simulink model "model2"  (R2022b)
settings: Solver=ode4  StartTime=0.0  StopTime=2  FixedStep=1e-5  RelTol=1e-3
InitFcn:
  | model_
values from neighbouring files (symbols this model uses):
  f = 50    [model_.m]
  J = 0.4    [model_.m]
  pp = 2    [model_.m]
undefined symbols (not defined in the file or in its folder): L1, L1sigma, L2, L2sigma, Lm, R1, R2, sigma
settings Model: Creator=petrzakopal  LastModifiedBy=petrzakopal

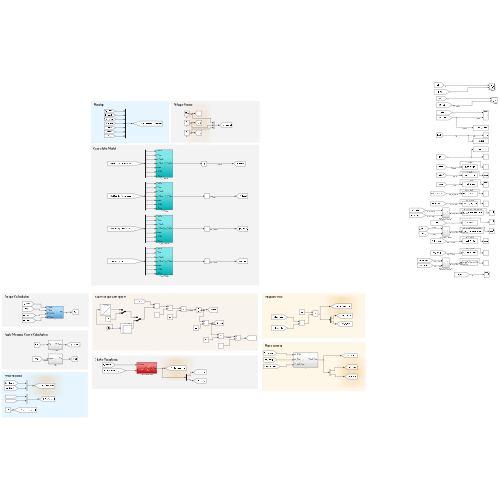
[thumbnail: Simulink's stored preview of the top-level diagram]
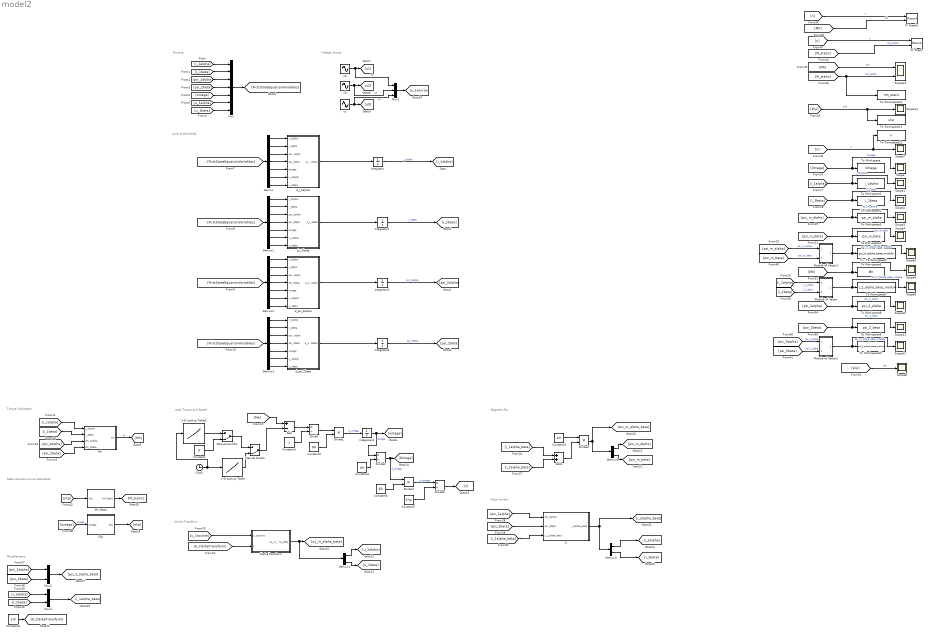
== system model2 ==
  note: Magnetic flux
  note: Rotor current
  note: Load Torque and Speed
  note: Clarke Transform
  note: Static Moment Curve Calculation
  note: Torque Calculation
  note: Core of the Model
  note: Miscellaneous
  note: Routing
  note: Voltage Source
  1-D Lookup Table : Lookup_n-D  NumberOfTableDimensions=1  BreakpointsForDimension1=[0;1.00001;1.001;10]  Table=[0;0;25;25]  InternalRulePriority=Speed  RndMeth=Simplest
  1-D Lookup Table2 : Lookup_n-D  NumberOfTableDimensions=1  BreakpointsForDimension1=[1;2;10]  Table=[0;0;78.48]  InternalRulePriority=Speed  RndMeth=Simplest
  Add : Sum  Inputs=+-
  Add1 : Sum
  ClarkeTransform : Subsystem
  Clock : Clock
  Constant : Constant  Value=0
  Constant1 : Constant  Value=J
  Constant2 : Constant  Value=pp
  Constant3 : Constant  Value=2/3
  Constant4 : Constant  Value=pp
  Constant5 : Constant  Value=Lm
  Constant6 : Constant  Value=60
  Constant7 : Constant  Value=2*pi
  Demux{,1..3} (4 alike) : Demux  Outputs=7
  Demux4 : Demux  Outputs=2
  Demux5 : Demux  Outputs=2
  Demux6 : Demux  Outputs=2
  Divide : Product  Inputs=*/
  Divide1 : Product  Inputs=**
  Divide2 : Product  Inputs=*/
  Divide3 : Product  Inputs=**
  Divide4 : Product  Inputs=**
  Divide5 : Product  Inputs=*/
  Integrator{,1..4} (5 alike) : Integrator
  Manual Switch : ManualSwitch  CurrentSetting=0
  Manual Switch1 : ManualSwitch  CurrentSetting=0
  Mh : Subsystem
  Mh Static : Subsystem
  Module of Vector : Subsystem
  Module of Vector1 : Subsystem
  Module of Vector2 : Subsystem
  Mux : Mux  Inputs=7
  Mux1 : Mux  Inputs=3
  Mux2 : Mux  Inputs=2
  Mux4 : Mux  Inputs=2
  Scope{,1..12,14} (14 alike) : Scope
  Scope13 : Scope  NumInputPorts=2
  Slip : Subsystem
  To Workspace : ToWorkspace  VariableName=Omega  SaveFormat=Timeseries  SampleTime=-1
  To Workspace1 : ToWorkspace  VariableName=i_1alpha  SaveFormat=Timeseries  SampleTime=-1
  To Workspace10 : ToWorkspace  VariableName=psi_2_alpha_beta_module  SaveFormat=Timeseries  SampleTime=-1
  To Workspace11 : ToWorkspace  VariableName=slip  SaveFormat=Timeseries  SampleTime=-1
  To Workspace12 : ToWorkspace  VariableName=mh_static  SaveFormat=Timeseries  SampleTime=-1
  To Workspace13 : ToWorkspace  VariableName=n  SaveFormat=Timeseries  SampleTime=-1
  To Workspace2 : ToWorkspace  VariableName=i_1beta  SaveFormat=Timeseries  SampleTime=-1
  To Workspace3 : ToWorkspace  VariableName=psi_m_alpha  SaveFormat=Timeseries  SampleTime=-1
  To Workspace4 : ToWorkspace  VariableName=psi_m_beta  SaveFormat=Timeseries  SampleTime=-1
  To Workspace5 : ToWorkspace  VariableName=psi_m_alpha_beta_module  SaveFormat=Timeseries  SampleTime=-1
  To Workspace6 : ToWorkspace  VariableName=Mh  SaveFormat=Timeseries  SampleTime=-1
  To Workspace7 : ToWorkspace  VariableName=i_1_alpha_beta_module  SaveFormat=Timeseries  SampleTime=-1
  To Workspace8 : ToWorkspace  VariableName=psi_2_alpha  SaveFormat=Timeseries  SampleTime=-1
  To Workspace9 : ToWorkspace  VariableName=psi_2_beta  SaveFormat=Timeseries  SampleTime=-1
  XY Graph : Record  FileSettingsInternal="{\"entries\":[{\"content\":{\"excelSettings\":{\"content\":{},\"type\":\"Streamout.ExcelSettings\"}},\"type\":\"Streamout.FileSettingStorage\",\"uuid\":\"842da89f-1fef-4ffd-8a1c-7bfb6317d6bb\"}],\"packageUris\":[\"http://schema.mathworks.com/mf0/streamout_blocks/R2020a\"],\"version\":\"1.0\"}"  Layout=[1 1]  SignalsInternal="{\"entries\":[{\"content\":{\"signals\":[{\"content\":{\"blockPath\":[\"model/XY Graph\"],\"channel\":[],\"dimensions\":[1],\"domain\":\"model/XY Graph\",\"lineColor\":\"#a2142f\",\"plots\":[1],\"port\":1,\"sid\":[],\"signalID\":16,\"signalName\":\"n\"},\"type\":\"RecordBlkView.Signal\",\"uuid\":\"3fa61c07-4d6e-48c9-97ec-bc673b73ea1e\"},{\"content\":{\"blockPath\":[\"model/XY Graph\"],\"channel\":[],\"dimensions\":[1],\"domain\":\"model/XY Graph\",\"lineColor\":\"#139fff\",\"plots\":[1],\"port\":2,\"sid\":[],\"signalID\":19,\"signalName\":\"Mh_static\"},\"type\":\"RecordBlkView.Signal\",\"uuid\":\"76ceb205-9b97-4673-bf6a-aa09134c6add\"}]},\"type\":\"RecordBlkView.InputSignals\",\"uuid\":\"48bfde53-39e3-4f40-beb6-cae9881eed94\"}],\"packageUris\":[\"http://schema.mathworks.com/mf0/streamout_blocks/R2020a\"],\"version\":\"1.0\"}"  VisualizationBindings="{\"xyplotplugin\":{\"info\":[{\"series\":[{\"bindingParametersList\":[{\"parameter\":\"X-Axis\",\"signalID\":16,\"signalName\":\"n\"},{\"parameter\":\"Y-Axis\",\"signalID\":19,\"signalName\":\"Mh_static\"}],\"seriesID\":25766}],\"subplotID\":1}]}}"  CompatibilityTag=XY
  XY Graph1 : Record  FileSettingsInternal="{\"entries\":[{\"content\":{\"excelSettings\":{\"content\":{},\"type\":\"Streamout.ExcelSettings\"}},\"type\":\"Streamout.FileSettingStorage\",\"uuid\":\"3db78ad4-fa90-443a-83a0-8f6baf93e8d6\"}],\"packageUris\":[\"http://schema.mathworks.com/mf0/streamout_blocks/R2020a\"],\"version\":\"1.0\"}"  Layout=[1 1]  SignalsInternal="{\"entries\":[{\"content\":{\"signals\":[{\"content\":{\"blockPath\":[\"model/XY Graph1\"],\"channel\":[],\"dimensions\":[1],\"domain\":\"model/XY Graph1\",\"lineColor\":\"#a2142f\",\"plots\":[1],\"port\":1,\"sid\":[],\"signalID\":8,\"signalName\":\"n\"},\"type\":\"RecordBlkView.Signal\",\"uuid\":\"17a0656e-17fb-4ce6-b629-ef989c268bcd\"},{\"content\":{\"blockPath\":[\"model/XY Graph1\"],\"channel\":[],\"dimensions\":[1],\"domain\":\"model/XY Graph1\",\"lineColor\":\"#139fff\",\"plots\":[1],\"port\":2,\"sid\":[],\"signalID\":11,\"signalName\":\"Mh\"},\"type\":\"RecordBlkView.Signal\",\"uuid\":\"9c618c76-db92-435b-920c-d0a40ae68f9d\"}]},\"type\":\"RecordBlkView.InputSignals\",\"uuid\":\"1549b7a0-6dc2-4283-9f7f-ab35875ee6b4\"}],\"packageUris\":[\"http://schema.mathworks.com/mf0/streamout_blocks/R2020a\"],\"version\":\"1.0\"}"  VisualizationBindings="{\"xyplotplugin\":{\"info\":[{\"series\":[{\"bindingParametersList\":[{\"parameter\":\"X-Axis\",\"signalID\":8,\"signalName\":\"n\"},{\"parameter\":\"Y-Axis\",\"signalID\":11,\"signalName\":\"Mh\"}],\"seriesID\":12463}],\"subplotID\":1}]}}"  CompatibilityTag=XY
  d_i_1alpha : Subsystem
  d_i_1beta : Subsystem
  d_psi_2alpha : Subsystem
  d_psi_2beta : Subsystem
  i2 : Subsystem
  ua : Sin  Amplitude=sqrt(2)*230  Frequency=2*pi*50  SampleTime=0
  ub : Sin  Amplitude=sqrt(2)*230  Frequency=2*pi*50  Phase=(2/3)*pi  SampleTime=0
  uc : Sin  Amplitude=sqrt(2)*230  Frequency=2*pi*50  Phase=-(2/3)*pi  SampleTime=0
  wires:
  Integrator/1 -> [i_1alpha]  "i_1alpha"
  Integrator1/1 -> [i_1beta]  "i_1beta"
  Integrator2/1 -> [psi_2alpha]  "psi_2alpha"
  Integrator3/1 -> [psi_2beta]  "psi_2beta"
  d_i_1alpha/1(d_i_1alpha) -> Integrator/1
  d_i_1beta/1(d_i_1beta) -> Integrator1/1
  [i_1alpha] -> Mux/1
  [i_1beta] -> Mux/2
  [psi_2alpha] -> Mux/3
  [psi_2beta] -> Mux/4
  [omega] -> Mux/5
  [u_1alpha] -> Mux/6
  [u_1beta] -> Mux/7
  Demux/1 -> d_i_1alpha/1(i_1alpha)
  Demux/2 -> d_i_1alpha/2(i_1beta)
  Demux/3 -> d_i_1alpha/3(psi_2alpha)
  Demux/4 -> d_i_1alpha/4(psi_2beta)
  Demux/5 -> d_i_1alpha/5(omega)
  Demux/6 -> d_i_1alpha/6(u_1alpha)
  Mux/1 -> [FirstStateEquationVariables]
  [FirstStateEquationVariables] -> Demux/1
  [FirstStateEquationVariables] -> Demux1/1
  Demux1/6 -> d_i_1beta/6(u_1alpha)
  Demux1/5 -> d_i_1beta/5(omega)
  Demux1/4 -> d_i_1beta/4(psi_2beta)
  Demux1/3 -> d_i_1beta/3(psi_2alpha)
  Demux1/2 -> d_i_1beta/2(i_1beta)
  Demux1/1 -> d_i_1beta/1(i_1alpha)
  Demux/7 -> d_i_1alpha/7(u_1beta)
  Demux1/7 -> d_i_1beta/7(u_1beta)
  Demux2/7 -> d_psi_2alpha/7(u_1beta)
  Demux2/1 -> d_psi_2alpha/1(i_1alpha)
  Demux2/2 -> d_psi_2alpha/2(i_1beta)
  Demux2/3 -> d_psi_2alpha/3(psi_2alpha)
  Demux2/4 -> d_psi_2alpha/4(psi_2beta)
  Demux2/5 -> d_psi_2alpha/5(omega)
  Demux2/6 -> d_psi_2alpha/6(u_1alpha)
  [FirstStateEquationVariables] -> Demux2/1
  d_psi_2alpha/1(d_psi_2alpha) -> Integrator2/1
  [FirstStateEquationVariables] -> Demux3/1
  Demux3/6 -> d_psi_2beta/6(u_1alpha)
  Demux3/5 -> d_psi_2beta/5(omega)
  Demux3/4 -> d_psi_2beta/4(psi_2beta)
  Demux3/3 -> d_psi_2beta/3(psi_2alpha)
  Demux3/7 -> d_psi_2beta/7(u_1beta)
  d_psi_2beta/1(d_psi_2beta) -> Integrator3/1
  Demux3/1 -> d_psi_2beta/1(i_1alpha)
  Demux3/2 -> d_psi_2beta/2(i_1beta)
  [i_1alpha] -> Mh/1(i_1alpha)
  [i_1beta] -> Mh/2(i_1beta)
  [psi_2alpha] -> Mh/3(phi_2alpha)
  [psi_2beta] -> Mh/4(phi_2beta)
  Mh/1(Mh) -> [Mh]  "M"
  [Mh] -> Add/1
  Clock/1 -> 1-D Lookup Table2/1, 1-D Lookup Table/1
  1-D Lookup Table/1 -> Manual Switch/2
  Manual Switch/1 -> Add/2
  Add/1 -> Divide/1
  Constant1/1 -> Divide/2
  Divide/1 -> Divide1/1
  Constant2/1 -> Divide1/2
  Divide1/1 -> Integrator4/1  "d_omega"
  Integrator4/1 -> Divide2/1, [omega]  "omega"
  ua/1 -> Mux1/1, [u1]  "ua"
  ub/1 -> Mux1/2, [u2]  "ub"
  uc/1 -> Mux1/3, [u3]  "uc"
  Mux1/1 -> [u_1source]
  Constant3/1 -> [K_ClarkeTransform]
  ClarkeTransform/1(u1_in_alpha_beta) -> Demux4/1, [u1_in_alpha_beta]
  [u_1source] -> ClarkeTransform/1(u_1source)
  [K_ClarkeTransform] -> ClarkeTransform/2(K)
  Demux4/1 -> [u_1alpha]
  Demux4/2 -> [u_1beta]
  Constant4/1 -> Divide2/2
  Divide2/1 -> Divide4/1, [Omega]  "d_omega"
  [Omega] -> Scope/1, To Workspace/1  "Omega"
  [i_1alpha] -> Scope1/1, To Workspace1/1  "I_1_alpha"
  [i_1beta] -> Scope2/1, To Workspace2/1  "i_1_beta"
  Constant5/1 -> Divide3/1
  Add1/1 -> Divide3/2
  [i_1alpha] -> Mux4/1
  [i_1beta] -> Mux4/2
  Mux4/1 -> [i_1alpha_beta]
  [i_1alpha_beta] -> Add1/1
  [i_2alpha_beta] -> Add1/2
  Divide3/1 -> Demux6/1, [psi_m_alpha_beta]
  Demux6/1 -> [psi_m_alpha]
  Demux6/2 -> [psi_m_beta]
  [psi_2alpha] -> i2/1(psi_2alpha)
  [psi_2beta] -> i2/2(psi_2beta)
  [i_1alpha_beta] -> i2/3(i_1_alpha_beta)
  i2/1(i_2alpha_beta) -> Demux5/1, [i_2alpha_beta]
  Demux5/1 -> [i_2alpha]
  Demux5/2 -> [i_2beta]
  [psi_m_alpha] -> Scope3/1, To Workspace3/1  "psi_m_alpha"
  [psi_m_beta] -> Scope4/1, To Workspace4/1  "psi_m_beta"
  Module of Vector1/1(Out1) -> Scope5/1, To Workspace5/1  "psi_m_alpha_beta_module"
  [Mh] -> Scope6/1, To Workspace6/1  "Mh"
  Constant6/1 -> Divide4/2
  Divide4/1 -> Divide5/1  "d_omega"
  Constant7/1 -> Divide5/2
  Divide5/1 -> [n]
  [n] -> To Workspace13/1, Scope7/1  "n"
  [psi_2alpha] -> Scope10/1, To Workspace8/1  "psi_2_alpha"
  [psi_2beta] -> To Workspace9/1, Scope11/1  "psi_2_beta"
  [psi_2alpha] -> Mux2/1
  [psi_2beta] -> Mux2/2
  Mux2/1 -> [psi_2_alpha_beta]
  [i_1alpha] -> Module of Vector/1(In1)  "I_1_alpha"
  [i_1beta] -> Module of Vector/2(In2)  "i_1_beta"
  [psi_m_alpha] -> Module of Vector1/1(In1)  "psi_m_alpha"
  [psi_m_beta] -> Module of Vector1/2(In2)  "psi_m_beta"
  Module of Vector/1(Out1) -> Scope9/1, To Workspace7/1  "psi_m_alpha_beta_module"
  Module of Vector2/1(Out1) -> Scope12/1, To Workspace10/1  "psi_m_alpha_beta_module"
  [psi_2alpha] -> Module of Vector2/1(In1)  "psi_2_alpha"
  [psi_2beta] -> Module of Vector2/2(In2)  "psi_2_beta"
  [slip] -> Mh Static/1(Slip)
  [Mh] -> Scope13/1  "Mh"
  [M_static] -> Scope13/2, To Workspace12/1  "Mh_static"
  Slip/1(Slip) -> [slip]
  Mh Static/1(Mh Static) -> [M_static]
  [slip] -> Scope14/1, To Workspace11/1  "slip"
  [M_static] -> XY Graph/2  "Mh_static"
  [n] -> XY Graph/1  "n"
  [omega] -> Slip/1(omega)  "omega"
  [n] -> XY Graph1/1  "n"
  [Mh] -> XY Graph1/2  "Mh"
  [slip] -> Scope8/1  "slip"
  1-D Lookup Table2/1 -> Manual Switch1/1
  Constant/1 -> Manual Switch1/2
  Manual Switch1/1 -> Manual Switch/1

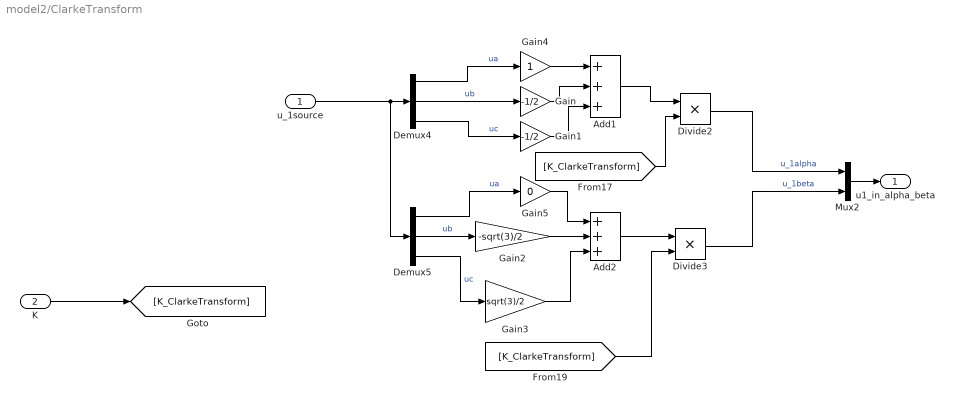
== system model2/ClarkeTransform ==
  u_1source : Inport
  K : Inport  Port=2
  Add1 : Sum  Inputs=+++
  Add2 : Sum  Inputs=+++
  Demux4 : Demux  Outputs=3
  Demux5 : Demux  Outputs=3
  Divide2 : Product  Inputs=**
  Divide3 : Product  Inputs=**
  Gain : Gain  Gain=-1/2
  Gain1 : Gain  Gain=-1/2
  Gain2 : Gain  Gain=-sqrt(3)/2
  Gain3 : Gain  Gain=sqrt(3)/2
  Gain4 : Gain
  Gain5 : Gain  Gain=0
  Mux2 : Mux  Inputs=2
  u1_in_alpha_beta : Outport
  wires:
  Demux4/1 -> Gain4/1  "ua"
  Divide2/1 -> Mux2/1  "u_1alpha"
  [K_ClarkeTransform] -> Divide2/2
  Add1/1 -> Divide2/1
  Demux4/2 -> Gain/1  "ub"
  Divide3/1 -> Mux2/2  "u_1beta"
  Gain5/1 -> Add2/1
  Gain/1 -> Add1/2
  Demux5/1 -> Gain5/1  "ua"
  Gain3/1 -> Add2/3
  [K_ClarkeTransform] -> Divide3/2
  Gain2/1 -> Add2/2
  Gain1/1 -> Add1/3
  Demux5/2 -> Gain2/1  "ub"
  Demux5/3 -> Gain3/1  "uc"
  Add2/1 -> Divide3/1
  Gain4/1 -> Add1/1
  u_1source/1 -> Demux5/1, Demux4/1
  K/1 -> [K_ClarkeTransform]
  Mux2/1 -> u1_in_alpha_beta/1
  Demux4/3 -> Gain1/1  "uc"

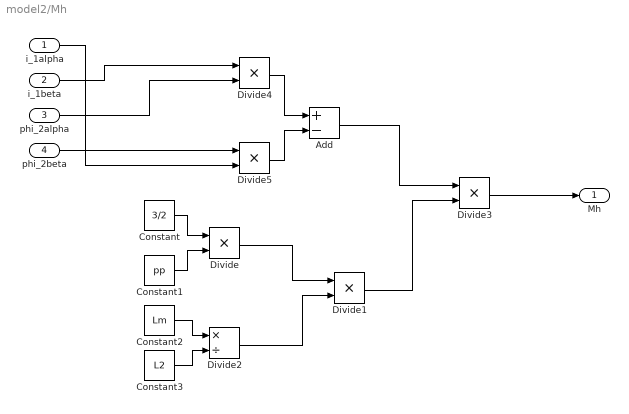
== system model2/Mh ==
  i_1alpha : Inport
  i_1beta : Inport  Port=2
  phi_2alpha : Inport  Port=3
  phi_2beta : Inport  Port=4
  Add : Sum  Inputs=+-
  Constant : Constant  Value=3/2
  Constant1 : Constant  Value=pp
  Constant2 : Constant  Value=Lm
  Constant3 : Constant  Value=L2
  Divide{,1,3..5} (5 alike) : Product  Inputs=**
  Divide2 : Product  Inputs=*/
  Mh : Outport
  wires:
  Constant/1 -> Divide/1
  Constant1/1 -> Divide/2
  Divide/1 -> Divide1/1
  Constant2/1 -> Divide2/1
  Constant3/1 -> Divide2/2
  Divide2/1 -> Divide1/2
  Divide1/1 -> Divide3/2
  phi_2alpha/1 -> Divide4/2
  i_1beta/1 -> Divide4/1
  Divide4/1 -> Add/1
  phi_2beta/1 -> Divide5/1
  i_1alpha/1 -> Divide5/2
  Divide5/1 -> Add/2
  Add/1 -> Divide3/1
  Divide3/1 -> Mh/1

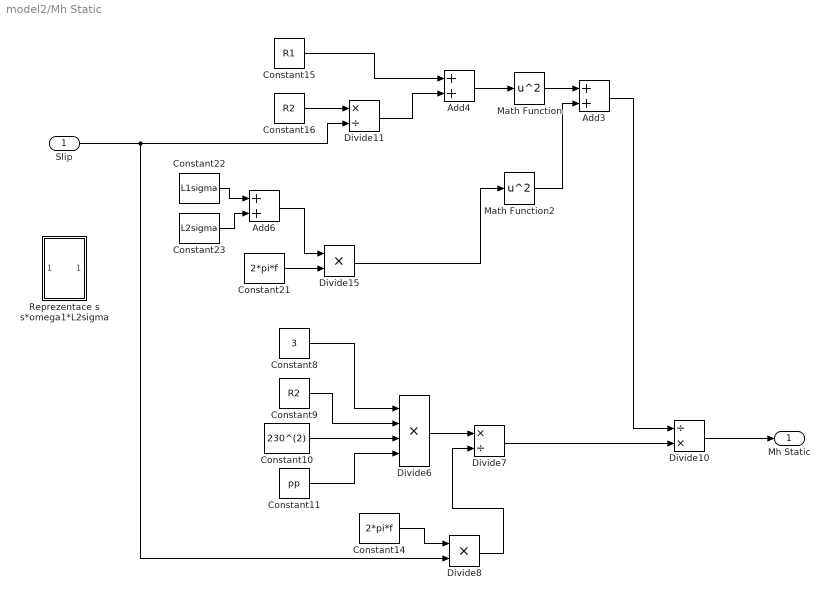
== system model2/Mh Static ==
  Slip : Inport
  Add3 : Sum
  Add4 : Sum
  Add6 : Sum
  Constant10 : Constant  Value=230^(2)
  Constant11 : Constant  Value=pp
  Constant14 : Constant  Value=2*pi*f
  Constant15 : Constant  Value=R1
  Constant16 : Constant  Value=R2
  Constant21 : Constant  Value=2*pi*f
  Constant22 : Constant  Value=L1sigma
  Constant23 : Constant  Value=L2sigma
  Constant8 : Constant  Value=3
  Constant9 : Constant  Value=R2
  Divide10 : Product  Inputs=/*
  Divide11 : Product  Inputs=*/
  Divide15 : Product  Inputs=**
  Divide6 : Product  Inputs=****
  Divide7 : Product  Inputs=*/
  Divide8 : Product  Inputs=**
  Math Function : Math  Operator=square
  Math Function2 : Math  Operator=square
  Reprezentace s s*omega1*L2sigma : Subsystem
  Mh Static : Outport
  wires:
  Slip/1 -> Divide8/2, Divide11/2
  Constant11/1 -> Divide6/4
  Constant10/1 -> Divide6/3
  Add4/1 -> Math Function/1
  Constant16/1 -> Divide11/1
  Constant9/1 -> Divide6/2
  Constant23/1 -> Add6/2
  Constant15/1 -> Add4/1
  Divide15/1 -> Math Function2/1
  Divide8/1 -> Divide7/2
  Constant14/1 -> Divide8/1
  Math Function/1 -> Add3/1
  Divide7/1 -> Divide10/2
  Divide10/1 -> Mh Static/1
  Divide11/1 -> Add4/2
  Constant22/1 -> Add6/1
  Add6/1 -> Divide15/1
  Constant8/1 -> Divide6/1
  Constant21/1 -> Divide15/2
  Add3/1 -> Divide10/1
  Divide6/1 -> Divide7/1
  Math Function2/1 -> Add3/2

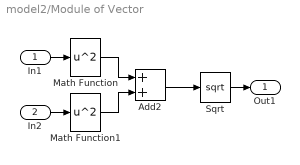
== system model2/Module of Vector ==
  In1 : Inport
  In2 : Inport  Port=2
  Add2 : Sum
  Math Function : Math  Operator=square
  Math Function1 : Math  Operator=square
  Sqrt : Sqrt
  Out1 : Outport
  wires:
  In1/1 -> Math Function/1
  Sqrt/1 -> Out1/1
  Math Function/1 -> Add2/1
  Math Function1/1 -> Add2/2
  In2/1 -> Math Function1/1
  Add2/1 -> Sqrt/1

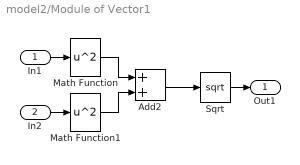
== system model2/Module of Vector1 ==
  In1 : Inport
  In2 : Inport  Port=2
  Add2 : Sum
  Math Function : Math  Operator=square
  Math Function1 : Math  Operator=square
  Sqrt : Sqrt
  Out1 : Outport
  wires:
  Add2/1 -> Sqrt/1
  In2/1 -> Math Function1/1
  Math Function1/1 -> Add2/2
  Math Function/1 -> Add2/1
  Sqrt/1 -> Out1/1
  In1/1 -> Math Function/1

== system model2/Module of Vector2 ==
  In1 : Inport
  In2 : Inport  Port=2
  Add2 : Sum
  Math Function : Math  Operator=square
  Math Function1 : Math  Operator=square
  Sqrt : Sqrt
  Out1 : Outport
  wires:
  Add2/1 -> Sqrt/1
  In2/1 -> Math Function1/1
  Math Function1/1 -> Add2/2
  Math Function/1 -> Add2/1
  Sqrt/1 -> Out1/1
  In1/1 -> Math Function/1

== system model2/Slip ==
  omega : Inport
  Add2 : Sum  Inputs=+-
  Constant12 : Constant  Value=2*pi*f
  Constant13 : Constant  Value=2*pi*f
  Divide9 : Product  Inputs=*/
  Slip : Outport
  wires:
  omega/1 -> Add2/2  "Omega"
  Divide9/1 -> Slip/1
  Constant12/1 -> Add2/1
  Add2/1 -> Divide9/1
  Constant13/1 -> Divide9/2

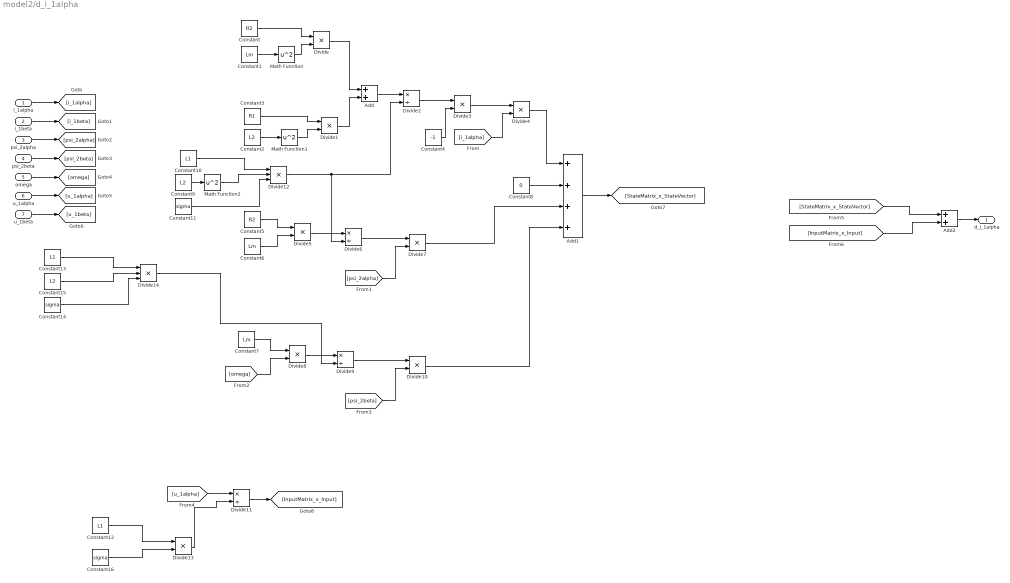
== system model2/d_i_1alpha ==
  i_1alpha : Inport
  i_1beta : Inport  Port=2
  psi_2alpha : Inport  Port=3
  psi_2beta : Inport  Port=4
  omega : Inport  Port=5
  u_1alpha : Inport  Port=6
  u_1beta : Inport  Port=7
  Add : Sum
  Add1 : Sum  Inputs=++++
  Add2 : Sum
  Constant : Constant  Value=R2
  Constant1 : Constant  Value=Lm
  Constant10 : Constant  Value=L1
  Constant11 : Constant  Value=sigma
  Constant12 : Constant  Value=L1
  Constant13 : Constant  Value=L1
  Constant14 : Constant  Value=sigma
  Constant15 : Constant  Value=L2
  Constant16 : Constant  Value=sigma
  Constant2 : Constant  Value=L2
  Constant3 : Constant  Value=R1
  Constant4 : Constant  Value=-1
  Constant5 : Constant  Value=R2
  Constant6 : Constant  Value=Lm
  Constant7 : Constant  Value=Lm
  Constant8 : Constant  Value=0
  Constant9 : Constant  Value=L2
  Divide{,1,3..5,7..8,10,13} (9 alike) : Product  Inputs=**
  Divide{2,6,9,11} (4 alike) : Product  Inputs=*/
  Divide12 : Product  Inputs=***
  Divide14 : Product  Inputs=***
  Math Function : Math  Operator=square
  Math Function1 : Math  Operator=square
  Math Function2 : Math  Operator=square
  d_i_1alpha : Outport
  wires:
  Constant1/1 -> Math Function/1
  Constant/1 -> Divide/1
  Math Function/1 -> Divide/2
  Divide/1 -> Add/1
  Constant2/1 -> Math Function1/1
  Constant3/1 -> Divide1/1
  Math Function1/1 -> Divide1/2
  Divide1/1 -> Add/2
  Add/1 -> Divide2/1
  Constant4/1 -> Divide3/2
  Divide2/1 -> Divide3/1
  Divide3/1 -> Divide4/1
  i_1alpha/1 -> [i_1alpha]
  i_1beta/1 -> [i_1beta]
  psi_2alpha/1 -> [psi_2alpha]
  psi_2beta/1 -> [psi_2beta]
  omega/1 -> [omega]
  [i_1alpha] -> Divide4/2
  Divide4/1 -> Add1/1
  Constant5/1 -> Divide5/1
  Constant6/1 -> Divide5/2
  Divide5/1 -> Divide6/1
  Divide6/1 -> Divide7/1
  [psi_2alpha] -> Divide7/2
  Divide7/1 -> Add1/3
  Constant7/1 -> Divide8/1
  [omega] -> Divide8/2
  Divide8/1 -> Divide9/1
  Divide9/1 -> Divide10/1
  [psi_2beta] -> Divide10/2
  Divide10/1 -> Add1/4
  Constant8/1 -> Add1/2
  u_1alpha/1 -> [u_1alpha]
  u_1beta/1 -> [u_1beta]
  Add1/1 -> [StateMatrix_x_StateVector]
  [u_1alpha] -> Divide11/1
  Divide11/1 -> [InputMatrix_x_Input]
  [StateMatrix_x_StateVector] -> Add2/1
  [InputMatrix_x_Input] -> Add2/2
  Add2/1 -> d_i_1alpha/1
  Constant9/1 -> Math Function2/1
  Constant10/1 -> Divide12/1
  Math Function2/1 -> Divide12/2
  Constant11/1 -> Divide12/3
  Divide12/1 -> Divide6/2, Divide2/2
  Constant14/1 -> Divide14/3
  Constant13/1 -> Divide14/1
  Constant15/1 -> Divide14/2
  Constant12/1 -> Divide13/1
  Constant16/1 -> Divide13/2
  Divide13/1 -> Divide11/2
  Divide14/1 -> Divide9/2

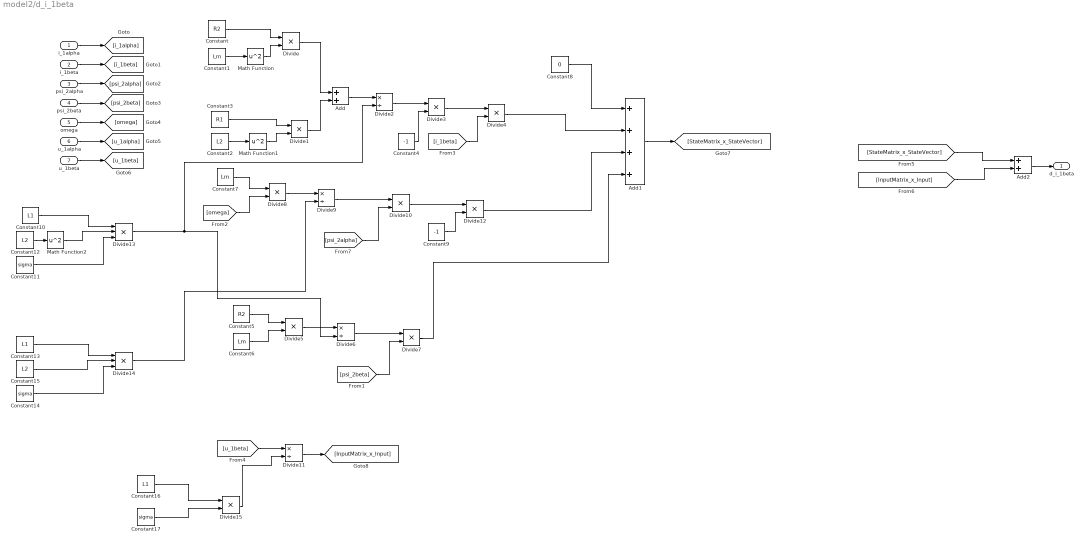
== system model2/d_i_1beta ==
  i_1alpha : Inport
  i_1beta : Inport  Port=2
  psi_2alpha : Inport  Port=3
  psi_2beta : Inport  Port=4
  omega : Inport  Port=5
  u_1alpha : Inport  Port=6
  u_1beta : Inport  Port=7
  Add : Sum
  Add1 : Sum  Inputs=++++
  Add2 : Sum
  Constant : Constant  Value=R2
  Constant1 : Constant  Value=Lm
  Constant10 : Constant  Value=L1
  Constant11 : Constant  Value=sigma
  Constant12 : Constant  Value=L2
  Constant13 : Constant  Value=L1
  Constant14 : Constant  Value=sigma
  Constant15 : Constant  Value=L2
  Constant16 : Constant  Value=L1
  Constant17 : Constant  Value=sigma
  Constant2 : Constant  Value=L2
  Constant3 : Constant  Value=R1
  Constant4 : Constant  Value=-1
  Constant5 : Constant  Value=R2
  Constant6 : Constant  Value=Lm
  Constant7 : Constant  Value=Lm
  Constant8 : Constant  Value=0
  Constant9 : Constant  Value=-1
  Divide{,1,3..5,7..8,10,12,15} (10 alike) : Product  Inputs=**
  Divide{2,6,9,11} (4 alike) : Product  Inputs=*/
  Divide13 : Product  Inputs=***
  Divide14 : Product  Inputs=***
  Math Function : Math  Operator=square
  Math Function1 : Math  Operator=square
  Math Function2 : Math  Operator=square
  d_i_1beta : Outport
  wires:
  Add2/1 -> d_i_1beta/1
  [InputMatrix_x_Input] -> Add2/2
  [StateMatrix_x_StateVector] -> Add2/1
  Divide11/1 -> [InputMatrix_x_Input]
  [u_1beta] -> Divide11/1
  Add1/1 -> [StateMatrix_x_StateVector]
  u_1beta/1 -> [u_1beta]
  u_1alpha/1 -> [u_1alpha]
  Constant8/1 -> Add1/1
  Divide10/1 -> Divide12/1
  [psi_2alpha] -> Divide10/2
  Divide9/1 -> Divide10/1
  Divide8/1 -> Divide9/1
  [omega] -> Divide8/2
  Constant7/1 -> Divide8/1
  Divide7/1 -> Add1/4
  [psi_2beta] -> Divide7/2
  Divide6/1 -> Divide7/1
  Divide5/1 -> Divide6/1
  Constant6/1 -> Divide5/2
  Constant5/1 -> Divide5/1
  Divide4/1 -> Add1/2
  [i_1beta] -> Divide4/2
  omega/1 -> [omega]
  psi_2beta/1 -> [psi_2beta]
  psi_2alpha/1 -> [psi_2alpha]
  i_1beta/1 -> [i_1beta]
  i_1alpha/1 -> [i_1alpha]
  Divide3/1 -> Divide4/1
  Divide2/1 -> Divide3/1
  Constant4/1 -> Divide3/2
  Add/1 -> Divide2/1
  Divide1/1 -> Add/2
  Math Function1/1 -> Divide1/2
  Constant3/1 -> Divide1/1
  Constant2/1 -> Math Function1/1
  Divide/1 -> Add/1
  Math Function/1 -> Divide/2
  Constant/1 -> Divide/1
  Constant1/1 -> Math Function/1
  Constant9/1 -> Divide12/2
  Divide12/1 -> Add1/3
  Constant10/1 -> Divide13/1
  Constant11/1 -> Divide13/3
  Math Function2/1 -> Divide13/2
  Divide13/1 -> Divide6/2, Divide2/2
  Constant12/1 -> Math Function2/1
  Divide14/1 -> Divide9/2
  Constant14/1 -> Divide14/3
  Constant15/1 -> Divide14/2
  Constant13/1 -> Divide14/1
  Constant16/1 -> Divide15/1
  Divide15/1 -> Divide11/2
  Constant17/1 -> Divide15/2

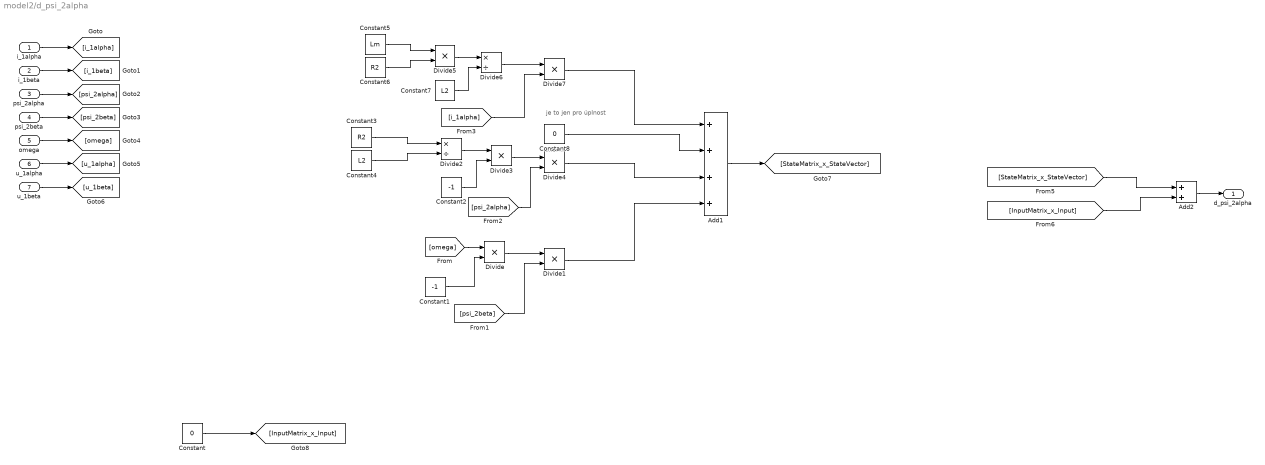
== system model2/d_psi_2alpha ==
  note: je to jen pro úplnost
  i_1alpha : Inport
  i_1beta : Inport  Port=2
  psi_2alpha : Inport  Port=3
  psi_2beta : Inport  Port=4
  omega : Inport  Port=5
  u_1alpha : Inport  Port=6
  u_1beta : Inport  Port=7
  Add1 : Sum  Inputs=++++
  Add2 : Sum
  Constant : Constant  Value=0
  Constant1 : Constant  Value=-1
  Constant2 : Constant  Value=-1
  Constant3 : Constant  Value=R2
  Constant4 : Constant  Value=L2
  Constant5 : Constant  Value=Lm
  Constant6 : Constant  Value=R2
  Constant7 : Constant  Value=L2
  Constant8 : Constant  Value=0
  Divide{,1,3..5,7} (6 alike) : Product  Inputs=**
  Divide2 : Product  Inputs=*/
  Divide6 : Product  Inputs=*/
  d_psi_2alpha : Outport
  wires:
  i_1alpha/1 -> [i_1alpha]
  i_1beta/1 -> [i_1beta]
  psi_2alpha/1 -> [psi_2alpha]
  psi_2beta/1 -> [psi_2beta]
  omega/1 -> [omega]
  Constant8/1 -> Add1/2
  u_1alpha/1 -> [u_1alpha]
  u_1beta/1 -> [u_1beta]
  Add1/1 -> [StateMatrix_x_StateVector]
  Constant/1 -> [InputMatrix_x_Input]
  [StateMatrix_x_StateVector] -> Add2/1
  [InputMatrix_x_Input] -> Add2/2
  Add2/1 -> d_psi_2alpha/1
  [omega] -> Divide/1
  Constant1/1 -> Divide/2
  Divide/1 -> Divide1/1
  [psi_2beta] -> Divide1/2
  Divide1/1 -> Add1/4
  Constant2/1 -> Divide3/2
  Divide2/1 -> Divide3/1
  Constant3/1 -> Divide2/1
  Constant4/1 -> Divide2/2
  Divide3/1 -> Divide4/1
  [psi_2alpha] -> Divide4/2
  Divide4/1 -> Add1/3
  Divide5/1 -> Divide6/1
  Constant5/1 -> Divide5/1
  Constant6/1 -> Divide5/2
  Constant7/1 -> Divide6/2
  Divide6/1 -> Divide7/1
  [i_1alpha] -> Divide7/2
  Divide7/1 -> Add1/1

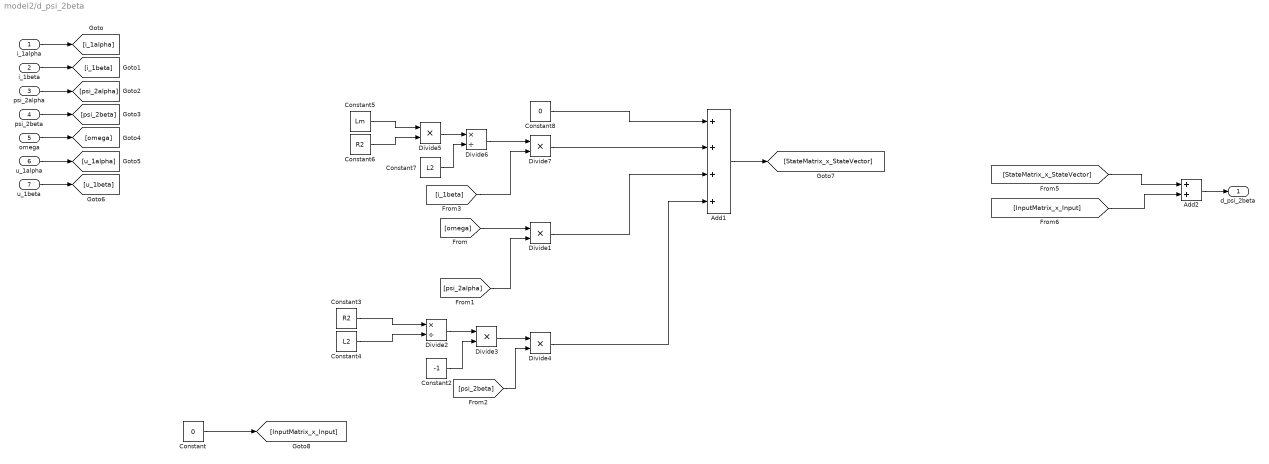
== system model2/d_psi_2beta ==
  i_1alpha : Inport
  i_1beta : Inport  Port=2
  psi_2alpha : Inport  Port=3
  psi_2beta : Inport  Port=4
  omega : Inport  Port=5
  u_1alpha : Inport  Port=6
  u_1beta : Inport  Port=7
  Add1 : Sum  Inputs=++++
  Add2 : Sum
  Constant : Constant  Value=0
  Constant2 : Constant  Value=-1
  Constant3 : Constant  Value=R2
  Constant4 : Constant  Value=L2
  Constant5 : Constant  Value=Lm
  Constant6 : Constant  Value=R2
  Constant7 : Constant  Value=L2
  Constant8 : Constant  Value=0
  Divide{1,3..5,7} (5 alike) : Product  Inputs=**
  Divide2 : Product  Inputs=*/
  Divide6 : Product  Inputs=*/
  d_psi_2beta : Outport
  wires:
  Divide7/1 -> Add1/2
  [i_1beta] -> Divide7/2
  Divide6/1 -> Divide7/1
  Constant7/1 -> Divide6/2
  Constant6/1 -> Divide5/2
  Constant5/1 -> Divide5/1
  Divide5/1 -> Divide6/1
  Divide4/1 -> Add1/4
  [psi_2beta] -> Divide4/2
  Divide3/1 -> Divide4/1
  Constant4/1 -> Divide2/2
  Constant3/1 -> Divide2/1
  Divide2/1 -> Divide3/1
  Constant2/1 -> Divide3/2
  Divide1/1 -> Add1/3
  [psi_2alpha] -> Divide1/2
  Add2/1 -> d_psi_2beta/1
  [InputMatrix_x_Input] -> Add2/2
  [StateMatrix_x_StateVector] -> Add2/1
  Constant/1 -> [InputMatrix_x_Input]
  Add1/1 -> [StateMatrix_x_StateVector]
  u_1beta/1 -> [u_1beta]
  u_1alpha/1 -> [u_1alpha]
  Constant8/1 -> Add1/1
  omega/1 -> [omega]
  psi_2beta/1 -> [psi_2beta]
  psi_2alpha/1 -> [psi_2alpha]
  i_1beta/1 -> [i_1beta]
  i_1alpha/1 -> [i_1alpha]
  [omega] -> Divide1/1

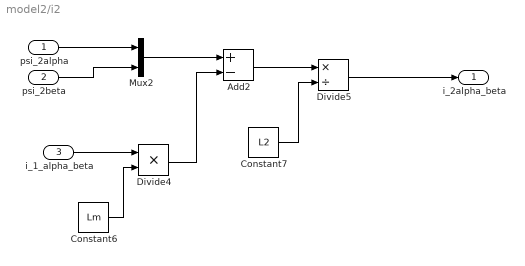
== system model2/i2 ==
  psi_2alpha : Inport
  psi_2beta : Inport  Port=2
  i_1_alpha_beta : Inport  Port=3
  Add2 : Sum  Inputs=+-
  Constant6 : Constant  Value=Lm
  Constant7 : Constant  Value=L2
  Divide4 : Product  Inputs=**
  Divide5 : Product  Inputs=*/
  Mux2 : Mux  Inputs=2
  i_2alpha_beta : Outport
  wires:
  psi_2alpha/1 -> Mux2/1
  Mux2/1 -> Add2/1
  Add2/1 -> Divide5/1
  Constant6/1 -> Divide4/2
  Divide4/1 -> Add2/2
  psi_2beta/1 -> Mux2/2
  Constant7/1 -> Divide5/2
  Divide5/1 -> i_2alpha_beta/1
  i_1_alpha_beta/1 -> Divide4/1

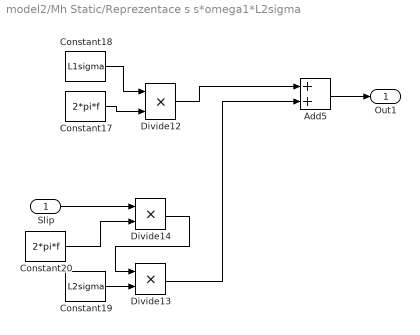
== system model2/Mh Static/Reprezentace s s*omega1*L2sigma ==
  Slip : Inport
  Add5 : Sum
  Constant17 : Constant  Value=2*pi*f
  Constant18 : Constant  Value=L1sigma
  Constant19 : Constant  Value=L2sigma
  Constant20 : Constant  Value=2*pi*f
  Divide12 : Product  Inputs=**
  Divide13 : Product  Inputs=**
  Divide14 : Product  Inputs=**
  Out1 : Outport
  wires:
  Divide13/1 -> Add5/2
  Divide14/1 -> Divide13/1
  Add5/1 -> Out1/1
  Constant18/1 -> Divide12/1
  Slip/1 -> Divide14/1
  Constant17/1 -> Divide12/2
  Divide12/1 -> Add5/1
  Constant20/1 -> Divide14/2
  Constant19/1 -> Divide13/2
